simulink model "DigitalCircuits"  (R2024b)
settings: Solver=FixedStepAuto  StartTime=0.0  StopTime=100  FixedStep=0.01  RelTol=1e-3
libraries: simulink_extras x6, simulink x2
settings Model: Creator=luigi  LastModifiedBy=luigi

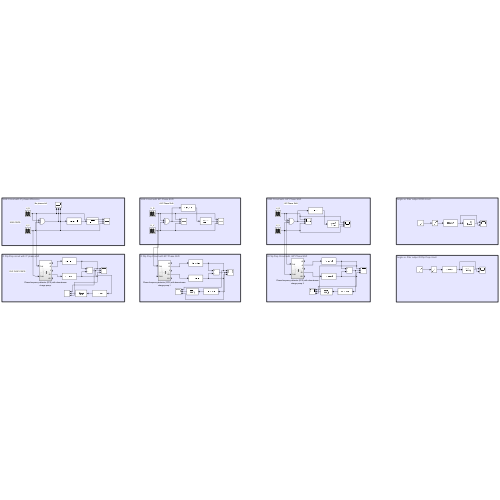
[thumbnail: Simulink's stored preview of the top-level diagram]
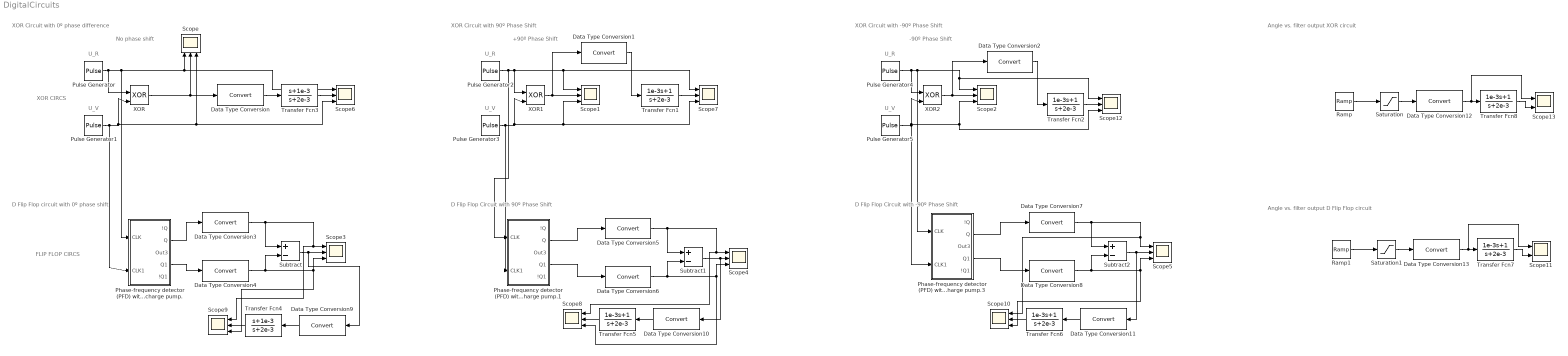
== system DigitalCircuits ==
  note: Angle vs. filter output D Flip Flop circuit
  note: Angle vs. filter output XOR circuit
  note: D Flip Flop Circuit with -90º Phase Shift
  note: XOR Circuit with -90º Phase Shift
  note: D Flip Flop Circuit with 90º Phase Shift
  note: XOR Circuit with 90º Phase Shift
  note: D Flip Flop circuit with 0º phase shift
  note: XOR Circuit with 0º phase difference
  note: FLIP FLOP CIRCS
  note: XOR CIRCS
  note: U_R
  note: No phase shift
  note: +90º Phase Shift
  note: -90º Phase Shift
  note: U_V
  note: U_R
  note: U_R
  note: U_V
  note: U_V
  Data Type Conversion{,1..13} (14 alike) : DataTypeConversion  SaturateOnIntegerOverflow=off  RndMeth=Floor
  Phase-frequency detector (PFD) with downstream charge pump. : Subsystem
  Phase-frequency detector (PFD) with downstream charge pump.1 : Subsystem
  Phase-frequency detector (PFD) with downstream charge pump.3 : Subsystem
  Pulse Generator : DiscretePulseGenerator  PulseType=Time based  Period=10  PulseWidth=50
  Pulse Generator1 : DiscretePulseGenerator  PulseType=Time based  Period=10  PulseWidth=50
  Pulse Generator2 : DiscretePulseGenerator  PulseType=Time based  Period=10  PulseWidth=50
  Pulse Generator3 : DiscretePulseGenerator  PulseType=Time based  Period=10  PulseWidth=50  PhaseDelay=2.5
  Pulse Generator4 : DiscretePulseGenerator  PulseType=Time based  Period=10  PulseWidth=5
  Pulse Generator5 : DiscretePulseGenerator  PulseType=Time based  Period=10  PulseWidth=5  PhaseDelay=-2.5
  Ramp : simulink/Sources/Ramp  slope=pi/50  start=0  InitialOutput=-pi
  Ramp1 : simulink/Sources/Ramp  slope=pi/100  start=0  InitialOutput=-pi/2
  Saturation : Saturate  UpperLimit=pi  LowerLimit=-pi
  Saturation1 : Saturate  UpperLimit=pi  LowerLimit=-pi
  Scope{,1..10,12} (12 alike) : Scope  NumInputPorts=3
  Scope11 : Scope  NumInputPorts=2
  Scope13 : Scope  NumInputPorts=2
  Subtract : Sum  Inputs=+-
  Subtract1 : Sum  Inputs=+-
  Subtract2 : Sum  Inputs=+-
  Transfer Fcn{1..2,5..8} (6 alike) : TransferFcn  Numerator=[1e-3 1]  Denominator=[1 2e-3]
  Transfer Fcn3 : TransferFcn  Numerator=[1 1e-3]  Denominator=[1 2e-3]
  Transfer Fcn4 : TransferFcn  Numerator=[1 1e-3]  Denominator=[1 2e-3]
  XOR : Logic  Operator=XOR  IconShape=distinctive  AllPortsSameDT=off  OutDataTypeStr=boolean
  XOR1 : Logic  Operator=XOR  IconShape=distinctive  AllPortsSameDT=off  OutDataTypeStr=boolean
  XOR2 : Logic  Operator=XOR  IconShape=distinctive  AllPortsSameDT=off  OutDataTypeStr=boolean
  wires:
  Pulse Generator1/1 -> Phase-frequency detector (PFD) with downstream charge pump./2(CLK1), Scope/3, Scope6/3, XOR/2
  Pulse Generator2/1 -> Phase-frequency detector (PFD) with downstream charge pump.1/1(CLK), Scope7/1, Scope1/1, XOR1/1
  XOR1/1 -> Data Type Conversion1/1, Scope1/2
  Pulse Generator3/1 -> Phase-frequency detector (PFD) with downstream charge pump.1/2(CLK1), Scope7/3, Scope1/3, XOR1/2
  XOR2/1 -> Data Type Conversion2/1, Scope2/2
  Pulse Generator/1 -> Scope6/1, Scope/1, Phase-frequency detector (PFD) with downstream charge pump./1(CLK), XOR/1
  XOR/1 -> Data Type Conversion/1, Scope/2
  Transfer Fcn3/1 -> Scope6/2
  Data Type Conversion/1 -> Transfer Fcn3/1
  Transfer Fcn1/1 -> Scope7/2
  Data Type Conversion1/1 -> Transfer Fcn1/1
  Transfer Fcn2/1 -> Scope12/2
  Data Type Conversion2/1 -> Transfer Fcn2/1
  Subtract/1 -> Data Type Conversion9/1, Scope3/2
  Phase-frequency detector (PFD) with downstream charge pump./2(Q) -> Data Type Conversion3/1
  Data Type Conversion3/1 -> Scope3/1, Scope9/1, Subtract/1
  Phase-frequency detector (PFD) with downstream charge pump./4(Q1) -> Data Type Conversion4/1
  Data Type Conversion4/1 -> Scope3/3, Scope9/3, Subtract/2
  Data Type Conversion6/1 -> Scope4/3, Scope8/3, Subtract1/2
  Data Type Conversion5/1 -> Scope4/1, Scope8/1, Subtract1/1
  Subtract1/1 -> Data Type Conversion10/1, Scope4/2
  Phase-frequency detector (PFD) with downstream charge pump.1/2(Q) -> Data Type Conversion5/1
  Phase-frequency detector (PFD) with downstream charge pump.1/4(Q1) -> Data Type Conversion6/1
  Subtract2/1 -> Data Type Conversion11/1, Scope5/2
  Data Type Conversion8/1 -> Scope10/3, Scope5/3, Subtract2/2
  Phase-frequency detector (PFD) with downstream charge pump.3/4(Q1) -> Data Type Conversion8/1
  Data Type Conversion7/1 -> Scope5/1, Scope10/1, Subtract2/1
  Phase-frequency detector (PFD) with downstream charge pump.3/2(Q) -> Data Type Conversion7/1
  Pulse Generator5/1 -> Phase-frequency detector (PFD) with downstream charge pump.3/2(CLK1), Scope2/3, Scope12/3, XOR2/2
  Pulse Generator4/1 -> Phase-frequency detector (PFD) with downstream charge pump.3/1(CLK), Scope12/1, Scope2/1, XOR2/1
  Transfer Fcn4/1 -> Scope9/2
  Data Type Conversion9/1 -> Transfer Fcn4/1
  Transfer Fcn5/1 -> Scope8/2
  Data Type Conversion10/1 -> Transfer Fcn5/1
  Transfer Fcn6/1 -> Scope10/2
  Data Type Conversion11/1 -> Transfer Fcn6/1
  Data Type Conversion12/1 -> Transfer Fcn8/1, Scope13/1
  Transfer Fcn8/1 -> Scope13/2
  Saturation/1 -> Data Type Conversion12/1
  Ramp/1 -> Saturation/1
  Saturation1/1 -> Data Type Conversion13/1
  Data Type Conversion13/1 -> Transfer Fcn7/1, Scope11/1
  Transfer Fcn7/1 -> Scope11/2
  Ramp1/1 -> Saturation1/1

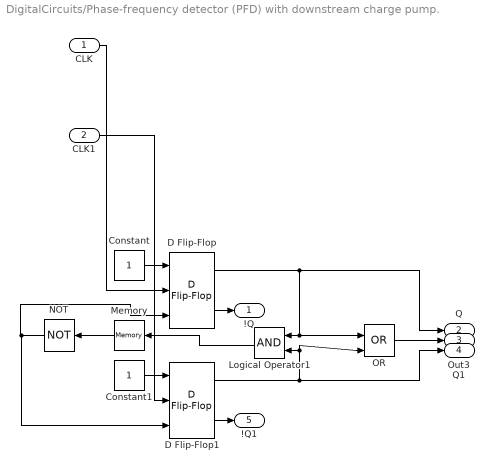
== system DigitalCircuits/Phase-frequency detector (PFD) with downstream charge pump. ==
  CLK : Inport
  CLK1 : Inport  Port=2
  Constant : Constant  OutDataTypeStr=boolean
  Constant1 : Constant  OutDataTypeStr=boolean
  D Flip-Flop : simulink_extras/Flip Flops/D Flip-Flop
  D Flip-Flop1 : simulink_extras/Flip Flops/D Flip-Flop
  Logical Operator1 : Logic  AllPortsSameDT=off  OutDataTypeStr=boolean
  Memory : Memory
  NOT : Logic  Operator=NOT  IconShape=distinctive  AllPortsSameDT=off  OutDataTypeStr=boolean
  OR : Logic  Operator=OR  IconShape=distinctive  AllPortsSameDT=off  OutDataTypeStr=boolean
  !Q : Outport
  Q : Outport  Port=2
  Out3 : Outport  Port=3
  Q1 : Outport  Port=4
  !Q1 : Outport  Port=5
  wires:
  Constant/1 -> D Flip-Flop/1
  Constant1/1 -> D Flip-Flop1/1
  D Flip-Flop/1 -> Q/1, OR/1, Logical Operator1/1
  OR/1 -> Out3/1
  D Flip-Flop1/1 -> Q1/1, OR/2, Logical Operator1/2
  Logical Operator1/1 -> Memory/1
  CLK/1 -> D Flip-Flop/2
  CLK1/1 -> D Flip-Flop1/2
  D Flip-Flop1/2 -> !Q1/1
  D Flip-Flop/2 -> !Q/1
  Memory/1 -> NOT/1
  NOT/1 -> D Flip-Flop1/3, D Flip-Flop/3

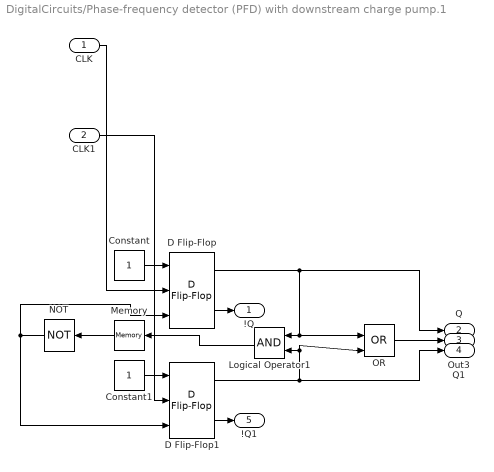
== system DigitalCircuits/Phase-frequency detector (PFD) with downstream charge pump.1 ==
  CLK : Inport
  CLK1 : Inport  Port=2
  Constant : Constant  OutDataTypeStr=boolean
  Constant1 : Constant  OutDataTypeStr=boolean
  D Flip-Flop : simulink_extras/Flip Flops/D Flip-Flop
  D Flip-Flop1 : simulink_extras/Flip Flops/D Flip-Flop
  Logical Operator1 : Logic  AllPortsSameDT=off  OutDataTypeStr=boolean
  Memory : Memory
  NOT : Logic  Operator=NOT  IconShape=distinctive  AllPortsSameDT=off  OutDataTypeStr=boolean
  OR : Logic  Operator=OR  IconShape=distinctive  AllPortsSameDT=off  OutDataTypeStr=boolean
  !Q : Outport
  Q : Outport  Port=2
  Out3 : Outport  Port=3
  Q1 : Outport  Port=4
  !Q1 : Outport  Port=5
  wires:
  Constant/1 -> D Flip-Flop/1
  Constant1/1 -> D Flip-Flop1/1
  D Flip-Flop/1 -> Q/1, OR/1, Logical Operator1/1
  OR/1 -> Out3/1
  D Flip-Flop1/1 -> Q1/1, OR/2, Logical Operator1/2
  Logical Operator1/1 -> Memory/1
  CLK/1 -> D Flip-Flop/2
  CLK1/1 -> D Flip-Flop1/2
  D Flip-Flop1/2 -> !Q1/1
  D Flip-Flop/2 -> !Q/1
  Memory/1 -> NOT/1
  NOT/1 -> D Flip-Flop1/3, D Flip-Flop/3

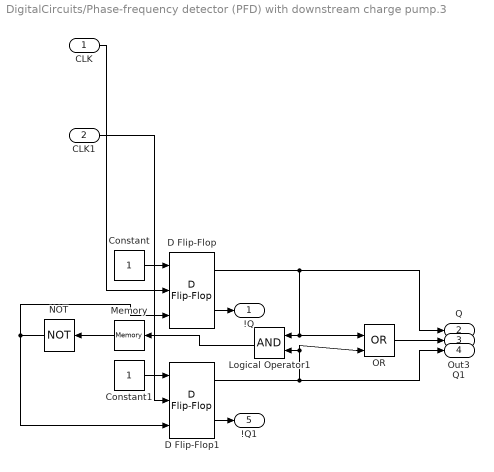
== system DigitalCircuits/Phase-frequency detector (PFD) with downstream charge pump.3 ==
  CLK : Inport
  CLK1 : Inport  Port=2
  Constant : Constant  OutDataTypeStr=boolean
  Constant1 : Constant  OutDataTypeStr=boolean
  D Flip-Flop : simulink_extras/Flip Flops/D Flip-Flop
  D Flip-Flop1 : simulink_extras/Flip Flops/D Flip-Flop
  Logical Operator1 : Logic  AllPortsSameDT=off  OutDataTypeStr=boolean
  Memory : Memory
  NOT : Logic  Operator=NOT  IconShape=distinctive  AllPortsSameDT=off  OutDataTypeStr=boolean
  OR : Logic  Operator=OR  IconShape=distinctive  AllPortsSameDT=off  OutDataTypeStr=boolean
  !Q : Outport
  Q : Outport  Port=2
  Out3 : Outport  Port=3
  Q1 : Outport  Port=4
  !Q1 : Outport  Port=5
  wires:
  Constant/1 -> D Flip-Flop/1
  Constant1/1 -> D Flip-Flop1/1
  D Flip-Flop/1 -> Q/1, OR/1, Logical Operator1/1
  OR/1 -> Out3/1
  D Flip-Flop1/1 -> Q1/1, OR/2, Logical Operator1/2
  Logical Operator1/1 -> Memory/1
  CLK/1 -> D Flip-Flop/2
  CLK1/1 -> D Flip-Flop1/2
  D Flip-Flop1/2 -> !Q1/1
  D Flip-Flop/2 -> !Q/1
  Memory/1 -> NOT/1
  NOT/1 -> D Flip-Flop1/3, D Flip-Flop/3
